simulink subsystem "motores"  (R2023b)
settings: Solver=VariableStepAuto  StartTime=0.0  StopTime=10.0  RelTol=1e-3
libraries: arduinolib x6, simulink x2
settings Model: Creator=Antonio  LastModifiedBy=Antonio

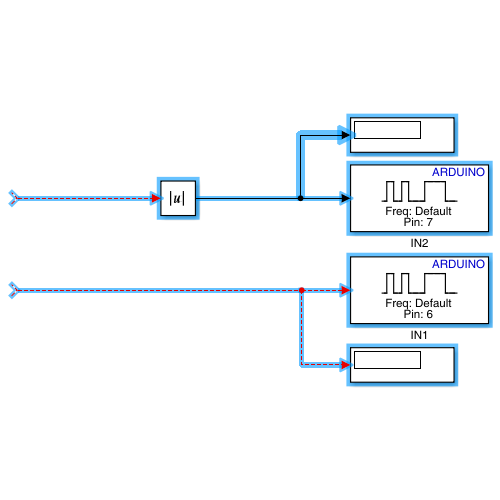
[thumbnail: Simulink's stored preview of the top-level diagram]
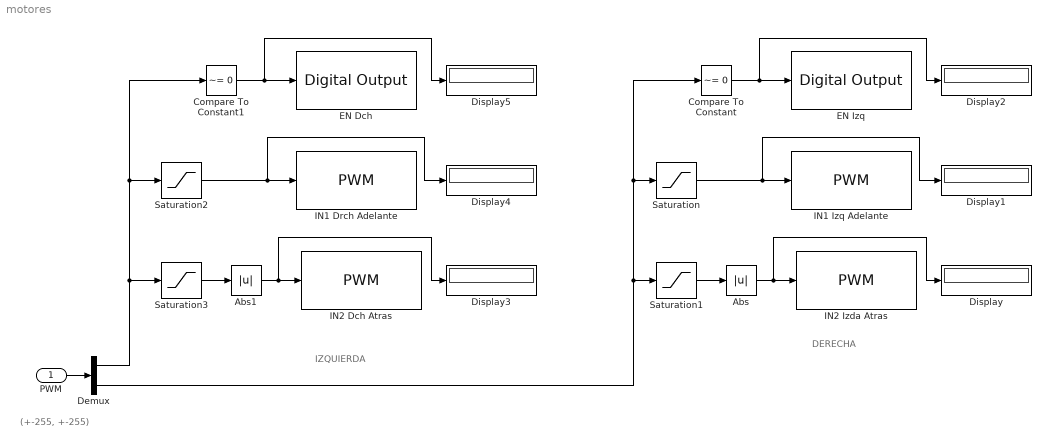
== system motores ==
  note: DERECHA
  note: IZQUIERDA
  note: (+-255, +-255)
  PWM : Inport
  Abs : Abs  SaturateOnIntegerOverflow=off
  Abs1 : Abs  SaturateOnIntegerOverflow=off
  Compare To Constant : simulink/Logic and Bit Operations/Compare To Constant  relop=~=  const=0  OutDataTypeStr=boolean
  Compare To Constant1 : simulink/Logic and Bit Operations/Compare To Constant  relop=~=  const=0  OutDataTypeStr=boolean
  Demux : Demux  Outputs=2
  Display{,1..5} (6 alike) : Display
  EN Dch : arduinolib/Digital Output  pinNumber=8  Direction=output  blockPlatform=arduino
  EN Izq : arduinolib/Digital Output  pinNumber=13  Direction=output  blockPlatform=arduino
  IN1 Drch Adelante : arduinolib/PWM  pinNumber=10  frequencyType=Default  desiredFrequency=490.2  achievableFrequency=490.2
  IN1 Izq Adelante : arduinolib/PWM  pinNumber=11  frequencyType=Default  desiredFrequency=490.2  achievableFrequency=490.2
  IN2 Dch Atras : arduinolib/PWM  pinNumber=9  frequencyType=Default  desiredFrequency=490.2  achievableFrequency=490.2
  IN2 Izda Atras : arduinolib/PWM  pinNumber=12  frequencyType=Default  desiredFrequency=490.2  achievableFrequency=490.2
  Saturation : Saturate  UpperLimit=255  LowerLimit=1
  Saturation1 : Saturate  UpperLimit=0  LowerLimit=-255
  Saturation2 : Saturate  UpperLimit=255  LowerLimit=1
  Saturation3 : Saturate  UpperLimit=0  LowerLimit=-255
  wires:
  Demux/2 -> Saturation1/1, Saturation/1, Compare To Constant/1
  Abs/1 -> Display/1, IN2 Izda Atras/1
  Compare To Constant/1 -> EN Izq/1, Display2/1
  Saturation/1 -> IN1 Izq Adelante/1, Display1/1
  Saturation1/1 -> Abs/1
  Saturation3/1 -> Abs1/1
  Saturation2/1 -> Display4/1, IN1 Drch Adelante/1
  Compare To Constant1/1 -> Display5/1, EN Dch/1
  Abs1/1 -> IN2 Dch Atras/1, Display3/1
  Demux/1 -> Saturation3/1, Compare To Constant1/1, Saturation2/1
  PWM/1 -> Demux/1
